simulink model "pasp_reordertest"  (Simulink 6.2)
settings: Solver=ode45  StartTime=0.0  StopTime=30000  RelTol=1e-3
undefined symbols (not defined in the file or in its folder): iBOB
libraries: xbsIndex_r3 x1464, casper_library x144, xps_library x60
(part 4 of 13)

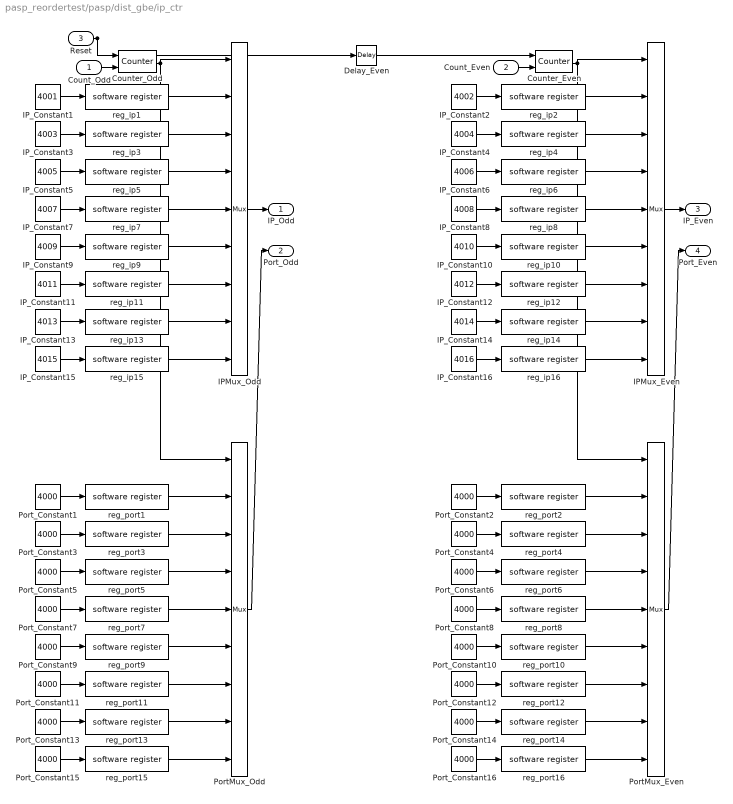
== system pasp_reordertest/pasp/dist_gbe/ip_ctr ==
  Count_Odd : Inport  Port=1  LatchInput=off
  Count_Even : Inport  Port=2  LatchInput=off
  Reset : Inport  Port=3  LatchInput=off
  Counter_Even : xbsIndex_r3/Counter  cnt_type=Free Running  n_bits=3  bin_pt=0  arith_type=Unsigned  start_count=0  cnt_to=Inf  cnt_by_val=1  operation=Up  explicit_period=off  period=1  load_pin=off  rst=on  en=on  dbl_ovrd=off  show_param=off  use_rpm=on  gen_core=off
      settings: xl_area=[0, 0, 0, 0, 0, 0, 0]
  Counter_Odd : xbsIndex_r3/Counter  cnt_type=Free Running  n_bits=3  bin_pt=0  arith_type=Unsigned  start_count=0  cnt_to=Inf  cnt_by_val=1  operation=Up  explicit_period=off  period=1  load_pin=off  rst=on  en=on  dbl_ovrd=off  show_param=off  use_rpm=on  gen_core=off
      settings: xl_area=[0, 0, 0, 0, 0, 0, 0]
  Delay_Even : xbsIndex_r3/Delay  latency=4  reg_retiming=off  explicit_period=off  period=1  en=off  accept_only_valid=off  init_zero=on  dbl_ovrd=off  show_param=off
      settings: xl_area=[0, 0, 0, 0, 0, 0, 0]
  IPMux_Even : xbsIndex_r3/Mux  inputs=8  precision=Full  arith_type="Signed  (2's comp)"  n_bits=8  bin_pt=2  quantization=Truncate  overflow=Wrap  latency=3  explicit_period=off  period=1  en=off  dbl_ovrd=off  show_param=off  mux_type=off  use_rpm=off  gen_core=off
      settings: xl_area=[0, 0, 0, 0, 0, 0, 0]
  IPMux_Odd : xbsIndex_r3/Mux  inputs=8  precision=Full  arith_type="Signed  (2's comp)"  n_bits=8  bin_pt=2  quantization=Truncate  overflow=Wrap  latency=3  explicit_period=off  period=1  en=off  dbl_ovrd=off  show_param=off  mux_type=off  use_rpm=off  gen_core=off
      settings: xl_area=[0, 0, 0, 0, 0, 0, 0]
  IP_Constant1 : Constant  Value=4001
  IP_Constant10 : Constant  Value=4010
  IP_Constant11 : Constant  Value=4011
  IP_Constant12 : Constant  Value=4012
  IP_Constant13 : Constant  Value=4013
  IP_Constant14 : Constant  Value=4014
  IP_Constant15 : Constant  Value=4015
  IP_Constant16 : Constant  Value=4016
  IP_Constant2 : Constant  Value=4002
  IP_Constant3 : Constant  Value=4003
  IP_Constant4 : Constant  Value=4004
  IP_Constant5 : Constant  Value=4005
  IP_Constant6 : Constant  Value=4006
  IP_Constant7 : Constant  Value=4007
  IP_Constant8 : Constant  Value=4008
  IP_Constant9 : Constant  Value=4009
  PortMux_Even : xbsIndex_r3/Mux  inputs=8  precision=Full  arith_type="Signed  (2's comp)"  n_bits=8  bin_pt=2  quantization=Truncate  overflow=Wrap  latency=3  explicit_period=off  period=1  en=off  dbl_ovrd=off  show_param=off  mux_type=off  use_rpm=off  gen_core=off
      settings: xl_area=[0, 0, 0, 0, 0, 0, 0]
  PortMux_Odd : xbsIndex_r3/Mux  inputs=8  precision=Full  arith_type="Signed  (2's comp)"  n_bits=8  bin_pt=2  quantization=Truncate  overflow=Wrap  latency=3  explicit_period=off  period=1  en=off  dbl_ovrd=off  show_param=off  mux_type=off  use_rpm=off  gen_core=off
      settings: xl_area=[0, 0, 0, 0, 0, 0, 0]
  Port_Constant{1..16} (16 alike) : Constant  Value=4000
  reg_ip1 : xps_library/software register  Tag=xps:sw_reg  io_dir=From Processor  arith_type=Unsigned  bitwidth=32  bin_pt=0  sample_period=1  gw_name=pasp_reordertest_pasp_dist_gbe_ip_ctr_reg_ip1_user_data_out
  reg_ip10 : xps_library/software register  Tag=xps:sw_reg  io_dir=From Processor  arith_type=Unsigned  bitwidth=32  bin_pt=0  sample_period=1  gw_name=pasp_reordertest_pasp_dist_gbe_ip_ctr_reg_ip10_user_data_out
  reg_ip11 : xps_library/software register  Tag=xps:sw_reg  io_dir=From Processor  arith_type=Unsigned  bitwidth=32  bin_pt=0  sample_period=1  gw_name=pasp_reordertest_pasp_dist_gbe_ip_ctr_reg_ip11_user_data_out
  reg_ip12 : xps_library/software register  Tag=xps:sw_reg  io_dir=From Processor  arith_type=Unsigned  bitwidth=32  bin_pt=0  sample_period=1  gw_name=pasp_reordertest_pasp_dist_gbe_ip_ctr_reg_ip12_user_data_out
  reg_ip13 : xps_library/software register  Tag=xps:sw_reg  io_dir=From Processor  arith_type=Unsigned  bitwidth=32  bin_pt=0  sample_period=1  gw_name=pasp_reordertest_pasp_dist_gbe_ip_ctr_reg_ip13_user_data_out
  reg_ip14 : xps_library/software register  Tag=xps:sw_reg  io_dir=From Processor  arith_type=Unsigned  bitwidth=32  bin_pt=0  sample_period=1  gw_name=pasp_reordertest_pasp_dist_gbe_ip_ctr_reg_ip14_user_data_out
  reg_ip15 : xps_library/software register  Tag=xps:sw_reg  io_dir=From Processor  arith_type=Unsigned  bitwidth=32  bin_pt=0  sample_period=1  gw_name=pasp_reordertest_pasp_dist_gbe_ip_ctr_reg_ip15_user_data_out
  reg_ip16 : xps_library/software register  Tag=xps:sw_reg  io_dir=From Processor  arith_type=Unsigned  bitwidth=32  bin_pt=0  sample_period=1  gw_name=pasp_reordertest_pasp_dist_gbe_ip_ctr_reg_ip16_user_data_out
  reg_ip2 : xps_library/software register  Tag=xps:sw_reg  io_dir=From Processor  arith_type=Unsigned  bitwidth=32  bin_pt=0  sample_period=1  gw_name=pasp_reordertest_pasp_dist_gbe_ip_ctr_reg_ip2_user_data_out
  reg_ip3 : xps_library/software register  Tag=xps:sw_reg  io_dir=From Processor  arith_type=Unsigned  bitwidth=32  bin_pt=0  sample_period=1  gw_name=pasp_reordertest_pasp_dist_gbe_ip_ctr_reg_ip3_user_data_out
  reg_ip4 : xps_library/software register  Tag=xps:sw_reg  io_dir=From Processor  arith_type=Unsigned  bitwidth=32  bin_pt=0  sample_period=1  gw_name=pasp_reordertest_pasp_dist_gbe_ip_ctr_reg_ip4_user_data_out
  reg_ip5 : xps_library/software register  Tag=xps:sw_reg  io_dir=From Processor  arith_type=Unsigned  bitwidth=32  bin_pt=0  sample_period=1  gw_name=pasp_reordertest_pasp_dist_gbe_ip_ctr_reg_ip5_user_data_out
  reg_ip6 : xps_library/software register  Tag=xps:sw_reg  io_dir=From Processor  arith_type=Unsigned  bitwidth=32  bin_pt=0  sample_period=1  gw_name=pasp_reordertest_pasp_dist_gbe_ip_ctr_reg_ip6_user_data_out
  reg_ip7 : xps_library/software register  Tag=xps:sw_reg  io_dir=From Processor  arith_type=Unsigned  bitwidth=32  bin_pt=0  sample_period=1  gw_name=pasp_reordertest_pasp_dist_gbe_ip_ctr_reg_ip7_user_data_out
  reg_ip8 : xps_library/software register  Tag=xps:sw_reg  io_dir=From Processor  arith_type=Unsigned  bitwidth=32  bin_pt=0  sample_period=1  gw_name=pasp_reordertest_pasp_dist_gbe_ip_ctr_reg_ip8_user_data_out
  reg_ip9 : xps_library/software register  Tag=xps:sw_reg  io_dir=From Processor  arith_type=Unsigned  bitwidth=32  bin_pt=0  sample_period=1  gw_name=pasp_reordertest_pasp_dist_gbe_ip_ctr_reg_ip9_user_data_out
  reg_port1 : xps_library/software register  Tag=xps:sw_reg  io_dir=From Processor  arith_type=Unsigned  bitwidth=32  bin_pt=0  sample_period=1  gw_name=pasp_reordertest_pasp_dist_gbe_ip_ctr_reg_port1_user_data_out
  reg_port10 : xps_library/software register  Tag=xps:sw_reg  io_dir=From Processor  arith_type=Unsigned  bitwidth=32  bin_pt=0  sample_period=1  gw_name=pasp_reordertest_pasp_dist_gbe_ip_ctr_reg_port10_user_data_out
  reg_port11 : xps_library/software register  Tag=xps:sw_reg  io_dir=From Processor  arith_type=Unsigned  bitwidth=32  bin_pt=0  sample_period=1  gw_name=pasp_reordertest_pasp_dist_gbe_ip_ctr_reg_port11_user_data_out
  reg_port12 : xps_library/software register  Tag=xps:sw_reg  io_dir=From Processor  arith_type=Unsigned  bitwidth=32  bin_pt=0  sample_period=1  gw_name=pasp_reordertest_pasp_dist_gbe_ip_ctr_reg_port12_user_data_out
  reg_port13 : xps_library/software register  Tag=xps:sw_reg  io_dir=From Processor  arith_type=Unsigned  bitwidth=32  bin_pt=0  sample_period=1  gw_name=pasp_reordertest_pasp_dist_gbe_ip_ctr_reg_port13_user_data_out
  reg_port14 : xps_library/software register  Tag=xps:sw_reg  io_dir=From Processor  arith_type=Unsigned  bitwidth=32  bin_pt=0  sample_period=1  gw_name=pasp_reordertest_pasp_dist_gbe_ip_ctr_reg_port14_user_data_out
  reg_port15 : xps_library/software register  Tag=xps:sw_reg  io_dir=From Processor  arith_type=Unsigned  bitwidth=32  bin_pt=0  sample_period=1  gw_name=pasp_reordertest_pasp_dist_gbe_ip_ctr_reg_port15_user_data_out
  reg_port16 : xps_library/software register  Tag=xps:sw_reg  io_dir=From Processor  arith_type=Unsigned  bitwidth=32  bin_pt=0  sample_period=1  gw_name=pasp_reordertest_pasp_dist_gbe_ip_ctr_reg_port16_user_data_out
  reg_port2 : xps_library/software register  Tag=xps:sw_reg  io_dir=From Processor  arith_type=Unsigned  bitwidth=32  bin_pt=0  sample_period=1  gw_name=pasp_reordertest_pasp_dist_gbe_ip_ctr_reg_port2_user_data_out
  reg_port3 : xps_library/software register  Tag=xps:sw_reg  io_dir=From Processor  arith_type=Unsigned  bitwidth=32  bin_pt=0  sample_period=1  gw_name=pasp_reordertest_pasp_dist_gbe_ip_ctr_reg_port3_user_data_out
  reg_port4 : xps_library/software register  Tag=xps:sw_reg  io_dir=From Processor  arith_type=Unsigned  bitwidth=32  bin_pt=0  sample_period=1  gw_name=pasp_reordertest_pasp_dist_gbe_ip_ctr_reg_port4_user_data_out
  reg_port5 : xps_library/software register  Tag=xps:sw_reg  io_dir=From Processor  arith_type=Unsigned  bitwidth=32  bin_pt=0  sample_period=1  gw_name=pasp_reordertest_pasp_dist_gbe_ip_ctr_reg_port5_user_data_out
  reg_port6 : xps_library/software register  Tag=xps:sw_reg  io_dir=From Processor  arith_type=Unsigned  bitwidth=32  bin_pt=0  sample_period=1  gw_name=pasp_reordertest_pasp_dist_gbe_ip_ctr_reg_port6_user_data_out
  reg_port7 : xps_library/software register  Tag=xps:sw_reg  io_dir=From Processor  arith_type=Unsigned  bitwidth=32  bin_pt=0  sample_period=1  gw_name=pasp_reordertest_pasp_dist_gbe_ip_ctr_reg_port7_user_data_out
  reg_port8 : xps_library/software register  Tag=xps:sw_reg  io_dir=From Processor  arith_type=Unsigned  bitwidth=32  bin_pt=0  sample_period=1  gw_name=pasp_reordertest_pasp_dist_gbe_ip_ctr_reg_port8_user_data_out
  reg_port9 : xps_library/software register  Tag=xps:sw_reg  io_dir=From Processor  arith_type=Unsigned  bitwidth=32  bin_pt=0  sample_period=1  gw_name=pasp_reordertest_pasp_dist_gbe_ip_ctr_reg_port9_user_data_out
  IP_Odd : Outport
  Port_Odd : Outport  Port=2
  IP_Even : Outport  Port=3
  Port_Even : Outport  Port=4
  wires:
  Reset/1 -> Counter_Odd/1, Delay_Even/1
  Count_Odd/1 -> Counter_Odd/2
  Counter_Odd/1 -> IPMux_Odd/1, PortMux_Odd/1
  IPMux_Odd/1 -> IP_Odd/1
  PortMux_Odd/1 -> Port_Odd/1
  Delay_Even/1 -> Counter_Even/1
  Count_Even/1 -> Counter_Even/2
  Counter_Even/1 -> IPMux_Even/1, PortMux_Even/1
  IPMux_Even/1 -> IP_Even/1
  PortMux_Even/1 -> Port_Even/1
  IP_Constant1/1 -> reg_ip1/1
  reg_ip1/1 -> IPMux_Odd/2
  Port_Constant1/1 -> reg_port1/1
  reg_port1/1 -> PortMux_Odd/2
  IP_Constant3/1 -> reg_ip3/1
  reg_ip3/1 -> IPMux_Odd/3
  Port_Constant3/1 -> reg_port3/1
  reg_port3/1 -> PortMux_Odd/3
  IP_Constant5/1 -> reg_ip5/1
  reg_ip5/1 -> IPMux_Odd/4
  Port_Constant5/1 -> reg_port5/1
  reg_port5/1 -> PortMux_Odd/4
  IP_Constant7/1 -> reg_ip7/1
  reg_ip7/1 -> IPMux_Odd/5
  Port_Constant7/1 -> reg_port7/1
  reg_port7/1 -> PortMux_Odd/5
  IP_Constant9/1 -> reg_ip9/1
  reg_ip9/1 -> IPMux_Odd/6
  Port_Constant9/1 -> reg_port9/1
  reg_port9/1 -> PortMux_Odd/6
  IP_Constant11/1 -> reg_ip11/1
  reg_ip11/1 -> IPMux_Odd/7
  Port_Constant11/1 -> reg_port11/1
  reg_port11/1 -> PortMux_Odd/7
  IP_Constant13/1 -> reg_ip13/1
  reg_ip13/1 -> IPMux_Odd/8
  Port_Constant13/1 -> reg_port13/1
  reg_port13/1 -> PortMux_Odd/8
  IP_Constant15/1 -> reg_ip15/1
  reg_ip15/1 -> IPMux_Odd/9
  Port_Constant15/1 -> reg_port15/1
  reg_port15/1 -> PortMux_Odd/9
  IP_Constant2/1 -> reg_ip2/1
  reg_ip2/1 -> IPMux_Even/2
  Port_Constant2/1 -> reg_port2/1
  reg_port2/1 -> PortMux_Even/2
  IP_Constant4/1 -> reg_ip4/1
  reg_ip4/1 -> IPMux_Even/3
  Port_Constant4/1 -> reg_port4/1
  reg_port4/1 -> PortMux_Even/3
  IP_Constant6/1 -> reg_ip6/1
  reg_ip6/1 -> IPMux_Even/4
  Port_Constant6/1 -> reg_port6/1
  reg_port6/1 -> PortMux_Even/4
  IP_Constant8/1 -> reg_ip8/1
  reg_ip8/1 -> IPMux_Even/5
  Port_Constant8/1 -> reg_port8/1
  reg_port8/1 -> PortMux_Even/5
  IP_Constant10/1 -> reg_ip10/1
  reg_ip10/1 -> IPMux_Even/6
  Port_Constant10/1 -> reg_port10/1
  reg_port10/1 -> PortMux_Even/6
  IP_Constant12/1 -> reg_ip12/1
  reg_ip12/1 -> IPMux_Even/7
  Port_Constant12/1 -> reg_port12/1
  reg_port12/1 -> PortMux_Even/7
  IP_Constant14/1 -> reg_ip14/1
  reg_ip14/1 -> IPMux_Even/8
  Port_Constant14/1 -> reg_port14/1
  reg_port14/1 -> PortMux_Even/8
  IP_Constant16/1 -> reg_ip16/1
  reg_ip16/1 -> IPMux_Even/9
  Port_Constant16/1 -> reg_port16/1
  reg_port16/1 -> PortMux_Even/9
